simulink model "SeguimientoTrayectorias"  (R2020b)
settings: Solver=ode3  StartTime=0.0  StopTime=100.0  FixedStep=Ts  RelTol=1e-3
values from neighbouring files (symbols this model uses):
  Ts = 100e-3    (= 0.1)    [ComparadorNARX.m]    (also in RunTrajectoryControl.m; TestBenchRun_Ej1.m; TestNARXRun.m; TestNARXRun_Ej2.m)
undefined symbols (not defined in the file or in its folder): DiscIntNeverNeededParam, sigbuilder_block
libraries: simulink x2
settings Model: Creator=patri  LastModifiedBy=Victor
settings DataIOCC: ReturnWorkspaceOutputs=off

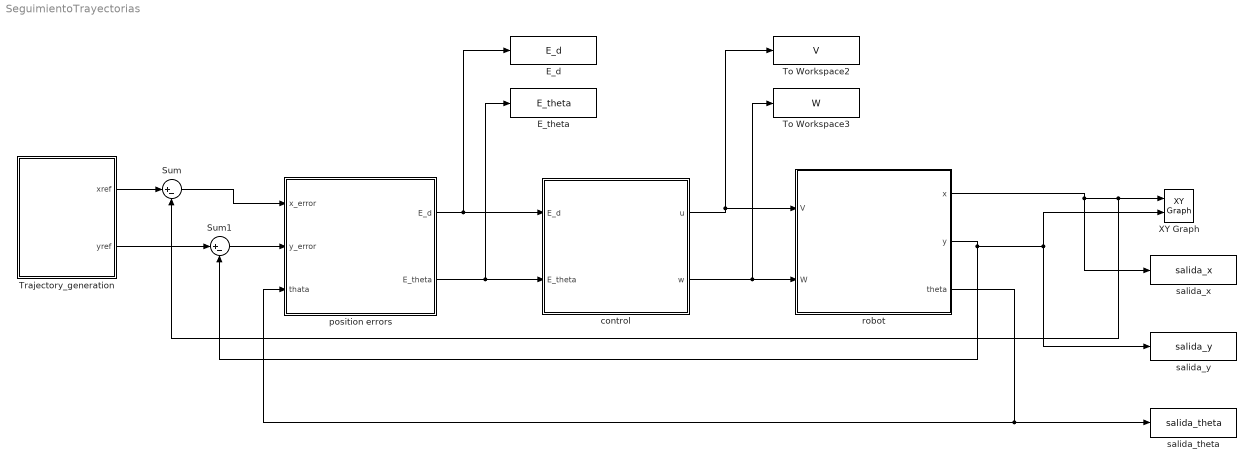
== system SeguimientoTrayectorias ==
  E_d : ToWorkspace  VariableName=E_d  SaveFormat=Structure With Time  SampleTime=-1
  E_theta : ToWorkspace  VariableName=E_theta  SaveFormat=Structure With Time  SampleTime=-1
  Sum : Sum  Inputs=|+-
  Sum1 : Sum  Inputs=|+-
  To Workspace2 : ToWorkspace  VariableName=V  SaveFormat=Structure With Time  SampleTime=-1
  To Workspace3 : ToWorkspace  VariableName=W  SaveFormat=Structure With Time  SampleTime=-1
  Trajectory_generation : Subsystem
  XY Graph : simulink/Sinks/XY Graph  xmin=-5  xmax=5  ymin=-5  ymax=5  st=-1
  control : Subsystem
  position errors : Subsystem
  robot : Subsystem
  salida_theta : ToWorkspace  VariableName=salida_theta  SaveFormat=Structure With Time  SampleTime=-1
  salida_x : ToWorkspace  VariableName=salida_x  SaveFormat=Structure With Time  SampleTime=-1
  salida_y : ToWorkspace  VariableName=salida_y  SaveFormat=Structure With Time  SampleTime=-1
  wires:
  control/1(u) -> To Workspace2/1, robot/1(V)
  position errors/1(E_d) -> control/1(E_d), E_d/1
  Sum1/1 -> position errors/2(y_error)
  Sum/1 -> position errors/1(x_error)
  Trajectory_generation/1(xref) -> Sum/1
  Trajectory_generation/2(yref) -> Sum1/1
  robot/1("x ") -> salida_x/1, Sum/2, XY Graph/1
  control/2(w) -> To Workspace3/1, robot/2("W ")
  robot/2(y) -> Sum1/2, salida_y/1, XY Graph/2
  robot/3(theta) -> position errors/3(thata), salida_theta/1
  position errors/2(E_theta) -> control/2(E_theta), E_theta/1

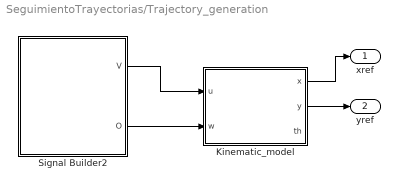
== system SeguimientoTrayectorias/Trajectory_generation ==
  Kinematic_model : Subsystem
  Signal Builder2 : Subsystem  Tag=STV Subsys  LoadFcn=sigbuilder_block('load');  StartFcn=sigbuilder_block('start');  StopFcn=sigbuilder_block('stop');  ClipboardFcn=sigbuilder_block('clipboard');  mask(Sigbuilder block){tuvar=[0:10]}
      mask help: Sigbuilder GUI
      mask init:
      | if ~strcmp(get_param(bdroot(gcbh),'SimulationStatus'),'stopped') tuvar = sigbuilder_block('maskInit'); end
      settings: CopyFcn=sigbuilder_block('copy');  DeleteFcn=sigbuilder_block('delete');  ModelCloseFcn=sigbuilder_block('modelClose');  PreSaveFcn=sigbuilder_block('preSave');  PauseFcn=sigbuilder_block('pause')  ContinueFcn=sigbuilder_block('continue')  NameChangeFcn=sigbuilder_block('namechange');  OpenFcn=sigbuilder_block('open',[60 82.4 534.4 508 ]);  CloseFcn=sigbuilder_block('close');
      mask Display: plot(0, 0, 100, 100,[2, 2, 32, 32, 2], [68, 8, 8, 68, 68],[32, 2], [38, 38], [32, 19, 2],[53, 60, 44], [32, 17, 17, 2],[16, 16, 31, 31]);txt = getActiveGroup(gcbh);text(2, 100, txt,'verticalAlignment', 'top');
  xref : Outport  VectorParamsAs1DForOutWhenUnconnected=off
  yref : Outport  Port=2  VectorParamsAs1DForOutWhenUnconnected=off
  wires:
  Signal Builder2/1(V) -> Kinematic_model/1(u)
  Signal Builder2/2(O) -> Kinematic_model/2(w)
  Kinematic_model/1(x) -> xref/1
  Kinematic_model/2(y) -> yref/1

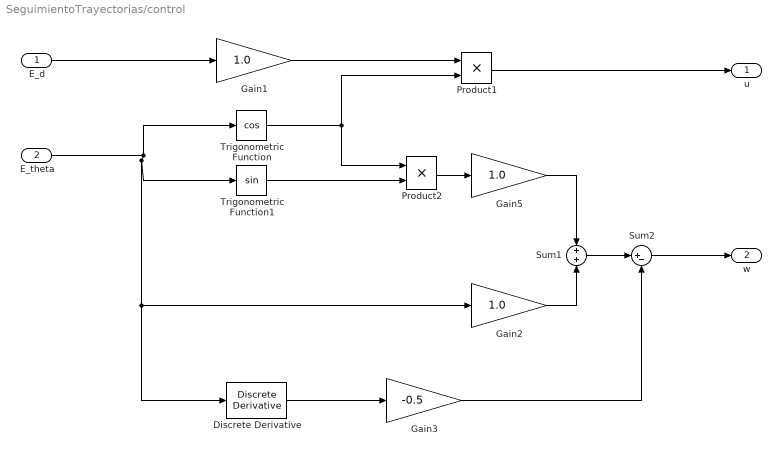
== system SeguimientoTrayectorias/control ==
  E_d : Inport
  E_theta : Inport  Port=2
  Discrete Derivative : simulink/Discrete/Discrete Derivative  gainval=1.0  ICPrevScaledInput=0.0  OutMin=[]  OutMax=[]  OutDataType=fixdt(1, 16)  OutScaling=2^-10  DoSatur=off
  Gain1 : Gain  Gain=1.0
  Gain2 : Gain  Gain=1.0
  Gain3 : Gain  Gain=-0.5
  Gain5 : Gain  Gain=1.0
  Product1 : Product
  Product2 : Product
  Sum1 : Sum
  Sum2 : Sum  Inputs=|+-
  Trigonometric Function : Trigonometry  Operator=cos
  Trigonometric Function1 : Trigonometry
  u : Outport  VectorParamsAs1DForOutWhenUnconnected=off
  w : Outport  Port=2  VectorParamsAs1DForOutWhenUnconnected=off
  wires:
  Product1/1 -> u/1
  Trigonometric Function/1 -> Product1/2, Product2/1
  Sum1/1 -> Sum2/1
  Gain3/1 -> Sum2/2
  Discrete Derivative/1 -> Gain3/1
  Sum2/1 -> w/1
  Product2/1 -> Gain5/1
  Gain1/1 -> Product1/1
  Gain2/1 -> Sum1/2
  Gain5/1 -> Sum1/1
  Trigonometric Function1/1 -> Product2/2
  E_d/1 -> Gain1/1
  E_theta/1 -> Trigonometric Function/1, Trigonometric Function1/1, Discrete Derivative/1, Gain2/1

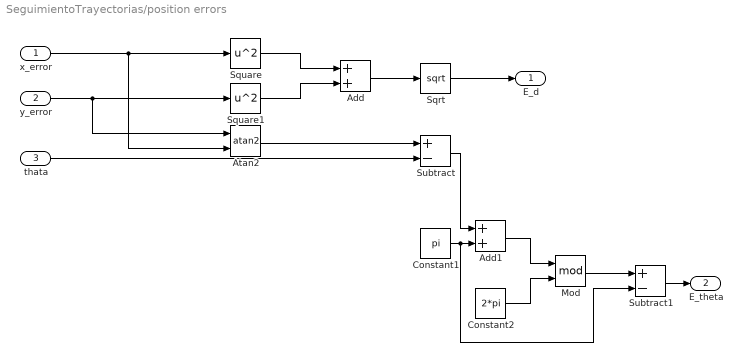
== system SeguimientoTrayectorias/position errors ==
  x_error : Inport  SampleTime=Ts
  y_error : Inport  Port=2  SampleTime=Ts
  thata : Inport  Port=3  SampleTime=Ts
  Add : Sum
  Add1 : Sum
  Atan2 : Trigonometry  Operator=atan2
  Constant1 : Constant  Value=pi  SampleTime=Ts
  Constant2 : Constant  Value=2*pi
  Mod : Math  Operator=mod  SignedPower=on  SaturateOnIntegerOverflow=on
  Sqrt : Sqrt  SaturateOnIntegerOverflow=on
  Square : Math  Operator=square  SignedPower=on  SaturateOnIntegerOverflow=on
  Square1 : Math  Operator=square  SignedPower=on  SaturateOnIntegerOverflow=on
  Subtract : Sum  Inputs=+-
  Subtract1 : Sum  Inputs=+-
  E_d : Outport  SampleTime=Ts  VectorParamsAs1DForOutWhenUnconnected=off
  E_theta : Outport  Port=2  SampleTime=Ts  VectorParamsAs1DForOutWhenUnconnected=off
  wires:
  x_error/1 -> Square/1, Atan2/2
  Square1/1 -> Add/2
  Atan2/1 -> Subtract/1
  Add1/1 -> Mod/1
  Subtract/1 -> Add1/1
  Mod/1 -> Subtract1/1
  Constant1/1 -> Subtract1/2, Add1/2
  y_error/1 -> Square1/1, Atan2/1
  Subtract1/1 -> E_theta/1
  Square/1 -> Add/1
  Constant2/1 -> Mod/2
  Sqrt/1 -> E_d/1
  thata/1 -> Subtract/2
  Add/1 -> Sqrt/1

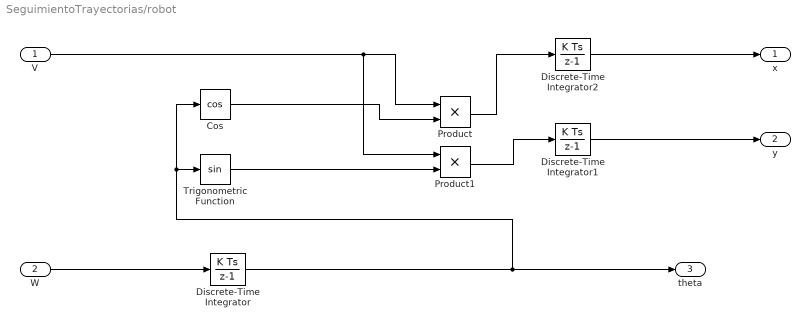
== system SeguimientoTrayectorias/robot ==
  V : Inport
  "W " : Inport  Port=2
  Cos : Trigonometry  Operator=cos
  Discrete-Time Integrator : DiscreteIntegrator  SampleTime=Ts  ICPrevOutput=DiscIntNeverNeededParam  ICPrevScaledInput=DiscIntNeverNeededParam
  Discrete-Time Integrator1 : DiscreteIntegrator  SampleTime=Ts  ICPrevOutput=DiscIntNeverNeededParam  ICPrevScaledInput=DiscIntNeverNeededParam
  Discrete-Time Integrator2 : DiscreteIntegrator  SampleTime=Ts  ICPrevOutput=DiscIntNeverNeededParam  ICPrevScaledInput=DiscIntNeverNeededParam
  Product : Product
  Product1 : Product
  Trigonometric Function : Trigonometry
  "x " : Outport
  y : Outport  Port=2
  theta : Outport  Port=3
  wires:
  Discrete-Time Integrator1/1 -> y/1
  "W "/1 -> Discrete-Time Integrator/1
  Trigonometric Function/1 -> Product1/2
  Product1/1 -> Discrete-Time Integrator1/1
  Discrete-Time Integrator2/1 -> "x "/1
  Product/1 -> Discrete-Time Integrator2/1
  Cos/1 -> Product/2
  V/1 -> Product1/1, Product/1
  Discrete-Time Integrator/1 -> theta/1, Cos/1, Trigonometric Function/1

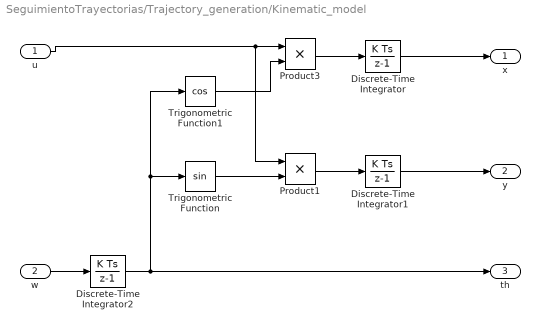
== system SeguimientoTrayectorias/Trajectory_generation/Kinematic_model ==
  u : Inport
  w : Inport  Port=2
  Discrete-Time Integrator : DiscreteIntegrator  SampleTime=Ts  ICPrevOutput=DiscIntNeverNeededParam  ICPrevScaledInput=DiscIntNeverNeededParam
  Discrete-Time Integrator1 : DiscreteIntegrator  SampleTime=Ts  ICPrevOutput=DiscIntNeverNeededParam  ICPrevScaledInput=DiscIntNeverNeededParam
  Discrete-Time Integrator2 : DiscreteIntegrator  SampleTime=Ts  ICPrevOutput=DiscIntNeverNeededParam  ICPrevScaledInput=DiscIntNeverNeededParam
  Product1 : Product
  Product3 : Product
  Trigonometric Function : Trigonometry
  Trigonometric Function1 : Trigonometry  Operator=cos
  x : Outport  VectorParamsAs1DForOutWhenUnconnected=off
  y : Outport  Port=2  VectorParamsAs1DForOutWhenUnconnected=off
  th : Outport  Port=3  VectorParamsAs1DForOutWhenUnconnected=off
  wires:
  Discrete-Time Integrator2/1 -> Trigonometric Function1/1, Trigonometric Function/1, th/1
  Product1/1 -> Discrete-Time Integrator1/1
  Product3/1 -> Discrete-Time Integrator/1
  w/1 -> Discrete-Time Integrator2/1
  Trigonometric Function/1 -> Product1/2
  u/1 -> Product1/1, Product3/1
  Trigonometric Function1/1 -> Product3/2
  Discrete-Time Integrator1/1 -> y/1
  Discrete-Time Integrator/1 -> x/1

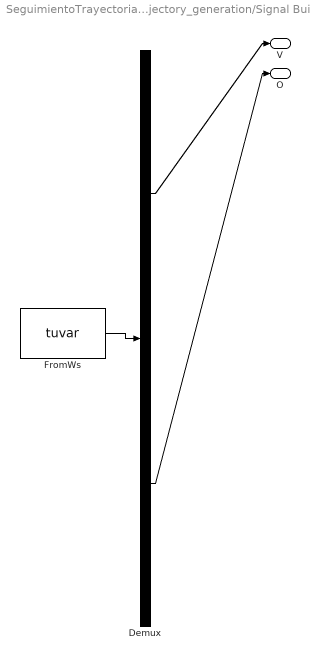
== system SeguimientoTrayectorias/Trajectory_generation/Signal Builder2 ==
  Demux : Demux  Tag=STV Demux  Outputs=2
      settings: DisplayOption=none
  FromWs : FromWorkspace  Tag=STV FromWs  VariableName=tuvar
      SigBuilderData=|
      | common.afterFinalStr = 'Extrapolate'
      | common.sampleTime = '0'
      | dataSet.timeRange = [0 115]
      | dataSet.name = 'Group 1'
      | sbobj.Groups.Name = 'Group 1'
      | sbobj.Groups.Signals(1).Name = 'V'
      | sbobj.Groups.Signals(1).XData = [0 87 87 115]
      | sbobj.Groups.Signals(1).YData = [0.25 0.25 0 0]
      | sbobj.Groups.Signals(2).Name = 'O'
      | sbobj.Groups.Signals(2).XData = [0 12 12 30.849 30.849 55.981 55.981 74.83 74.83 99.962 115]
      | sbobj.Groups.Signals(2).YData = [0 0 0.25 0.25 -0.25 -0.25 0.25 0.25 0 0 0]
      | sbobj.Groups.TimeRange = [0 115]
  V : Outport  Tag=STV Outport  VectorParamsAs1DForOutWhenUnconnected=off
  O : Outport  Tag=STV Outport  Port=2  VectorParamsAs1DForOutWhenUnconnected=off
  wires:
  FromWs/1 -> Demux/1
  Demux/1 -> V/1
  Demux/2 -> O/1
